simulink model "Simulation4"  (R2023b)
settings: Solver=VariableStepAuto  StartTime=0.0  StopTime=2  RelTol=1e-3
settings Model: Creator=vande_2  LastModifiedBy=vande_2

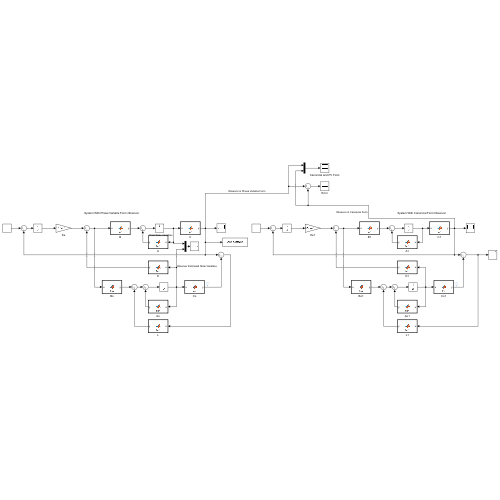
[thumbnail: Simulink's stored preview of the top-level diagram]
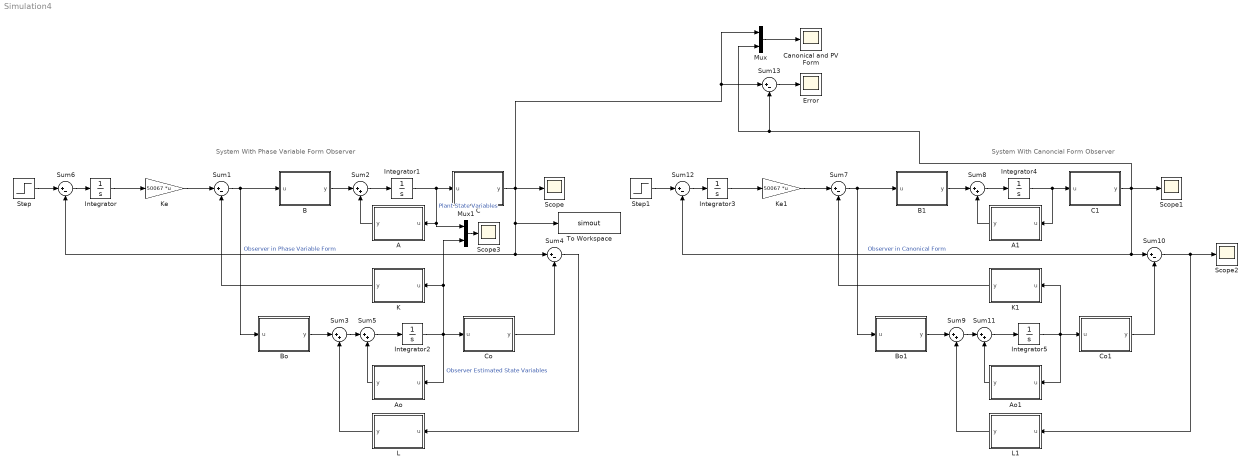
== system Simulation4 ==
  note: System With Phase Variable Form Observer
  note: System With Canoncial Form Observer
  A : MATLAB Function  TreatAsAtomicUnit=on
  A1 : MATLAB Function  TreatAsAtomicUnit=on
  Ao : MATLAB Function  TreatAsAtomicUnit=on
  Ao1 : MATLAB Function  TreatAsAtomicUnit=on
  B : MATLAB Function  TreatAsAtomicUnit=on
  B1 : MATLAB Function  TreatAsAtomicUnit=on
  Bo : MATLAB Function  TreatAsAtomicUnit=on
  Bo1 : MATLAB Function  TreatAsAtomicUnit=on
  C : MATLAB Function  TreatAsAtomicUnit=on
  C1 : MATLAB Function  TreatAsAtomicUnit=on
  Canonical and PV Form : Scope
  Co : MATLAB Function  TreatAsAtomicUnit=on
  Co1 : MATLAB Function  TreatAsAtomicUnit=on
  Error : Scope
  Integrator{,1,3..4} (4 alike) : Integrator
  Integrator2 : Integrator  InitialCondition=[2; 2]
  Integrator5 : Integrator  InitialCondition=[2; 2]
  K : MATLAB Function  TreatAsAtomicUnit=on
  K1 : MATLAB Function  TreatAsAtomicUnit=on
  Ke : Gain  Gain=50067  Multiplication=Matrix(K*u) (u vector)
  Ke1 : Gain  Gain=50067  Multiplication=Matrix(K*u) (u vector)
  L : MATLAB Function  TreatAsAtomicUnit=on
  L1 : MATLAB Function  TreatAsAtomicUnit=on
  Mux : Mux  Inputs=2
  Mux1 : Mux  Inputs=2
  Scope{,1..3} (4 alike) : Scope
  Step : Step  Time=0  SampleTime=0
  Step1 : Step  Time=0  SampleTime=0
  Sum{1,4,6..7,10,12..13} (7 alike) : Sum  Inputs=|+-
  Sum{2..3,5,8..9,11} (6 alike) : Sum  Inputs=|++
  To Workspace : ToWorkspace  VariableName=simout  SaveFormat=Timeseries  SampleTime=-1
  wires:
  B/1(y) -> Sum2/1
  Sum2/1 -> Integrator1/1
  Bo/1(y) -> Sum3/1
  Sum5/1 -> Integrator2/1
  Integrator2/1 -> Co/1(u), Mux1/2, K/1(u), Ao/1(u)  "Observer Estimated State Variables"
  Sum4/1 -> L/1(u)
  Integrator1/1 -> Mux1/1, A/1(u), C/1(u)  "Plant State Variables"
  A/1(y) -> Sum2/2
  Ao/1(y) -> Sum5/2
  L/1(y) -> Sum3/2
  Step/1 -> Sum6/1
  Co/1(y) -> Sum4/2
  Sum3/1 -> Sum5/1
  Sum6/1 -> Integrator/1
  Integrator/1 -> Ke/1
  Ke/1 -> Sum1/1
  Sum1/1 -> Bo/1(u), B/1(u)
  K/1(y) -> Sum1/2
  Co1/1(y) -> Sum10/2
  L1/1(y) -> Sum9/2
  K1/1(y) -> Sum7/2
  Sum7/1 -> Bo1/1(u), B1/1(u)
  Integrator5/1 -> Co1/1(u), K1/1(u), Ao1/1(u)
  Sum11/1 -> Integrator5/1
  Ke1/1 -> Sum7/1
  Integrator3/1 -> Ke1/1
  Ao1/1(y) -> Sum11/2
  Sum10/1 -> Scope2/1, L1/1(u)
  Sum9/1 -> Sum11/1
  Sum12/1 -> Integrator3/1
  Step1/1 -> Sum12/1
  A1/1(y) -> Sum8/2
  Sum8/1 -> Integrator4/1
  B1/1(y) -> Sum8/1
  Bo1/1(y) -> Sum9/1
  Integrator4/1 -> A1/1(u), C1/1(u)
  Mux/1 -> Canonical and PV Form/1
  Sum13/1 -> Error/1
  C/1(y) -> Sum13/1, Mux/1, Scope/1, Sum4/1, Sum6/2, To Workspace/1  "Observer in Phase Variable Form"
  C1/1(y) -> Sum13/2, Mux/2, Scope1/1, Sum10/1, Sum12/2  "Observer in Canonical Form"
  Mux1/1 -> Scope3/1

== matlab function Simulation4/K1 ==
  data: u input; y output
function y = fcn(u)
K = [418.169 47.4304];
y = K*u;

== matlab function Simulation4/L1 ==
  data: u input; y output
function y = fcn(u)
L = [1012.755;  125174.327];
y = L*u;

== matlab function Simulation4/Ao ==
  data: u input; y output
function y = fcn(u)
A = [0 1; 0 -0.5696];
y = A*u;

== matlab function Simulation4/B ==
  data: u input; y output
function y = fcn(u)
B = [0; 1];
y = B*u;

== matlab function Simulation4/C ==
  data: u input; y output
function y = fcn(u)
C = [0.07843, 0];
y = C*u;

== matlab function Simulation4/Bo ==
  data: u input; y output
function y = fcn(u)
B = [0; 1];
y = B*u;

== matlab function Simulation4/Co ==
  data: u input; y output
function y = fcn(u)
C = [0.0784 0];
y = C*u;

== matlab function Simulation4/L ==
  data: u input; y output
function y = fcn(u)
L = [1012.755;  125174.327];
y = L*u;

== matlab function Simulation4/K ==
  data: u input; y output
function y = fcn(u)
K = [418.169 47.4304];
y = K*u;

== matlab function Simulation4/A1 ==
  data: u input; y output
function y = fcn(u)
A = [0 1; 0 -0.5696];
y = A*u;

== matlab function Simulation4/A ==
  data: u input; y output
function y = fcn(u)
A = [0 1; 0 -0.5696];
y = A*u;

== matlab function Simulation4/Ao1 ==
  data: u input; y output
function y = fcn(u)
A = [-0.5696 1; 0 0];
y = A*u;

== matlab function Simulation4/B1 ==
  data: u input; y output
function y = fcn(u)
B = [0; 1];
y = B*u;

== matlab function Simulation4/Bo1 ==
  data: u input; y output
function y = fcn(u)
B = [0; 0.0784];
y = B*u;

== matlab function Simulation4/C1 ==
  data: u input; y output
function y = fcn(u)
C = [0.07843, 0];
y = C*u;

== matlab function Simulation4/Co1 ==
  data: u input; y output
function y = fcn(u)
C = [1 0];
y = C*u;
